simulink model "Project_Automotive_Performance_Modes"  (R2023a)
settings: Solver=VariableStepAuto  StartTime=0.0  StopTime=10.0  RelTol=1e-3
libraries: simulink x3, SignalEditorBlockLib x1
settings Model: Creator=Aman  LastModifiedBy=Aman

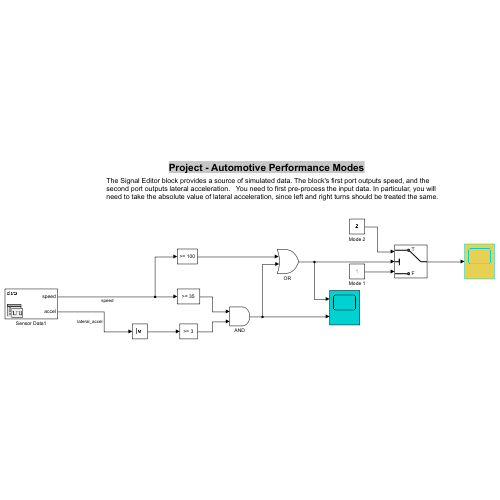
[thumbnail: Simulink's stored preview of the top-level diagram]
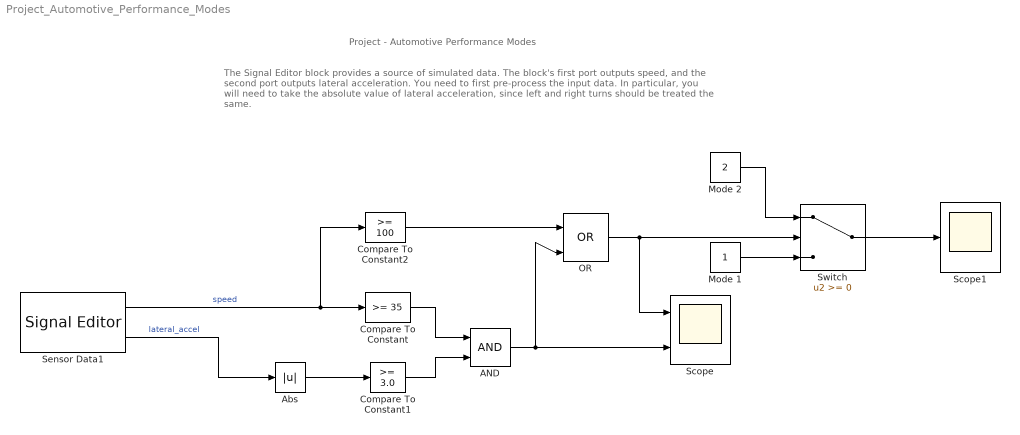
== system Project_Automotive_Performance_Modes ==
  note: The Signal Editor block provides a source of simulated data. The block's first port outputs speed, and the second port outputs lateral acceleration. You need to first pre-process the input data. In particular, you will need to take the absolute value of lateral acceleration, since left and right turns should be treated the same.
  note: Project - Automotive Performance Modes
  AND : Logic  IconShape=distinctive  AllPortsSameDT=off  OutDataTypeStr=boolean
  Abs : Abs  SaturateOnIntegerOverflow=off
  Compare To Constant : simulink/Logic and Bit Operations/Compare To Constant  relop=>=  const=35  OutDataTypeStr=boolean
  Compare To Constant1 : simulink/Logic and Bit Operations/Compare To Constant  relop=>=  const=3.0  OutDataTypeStr=boolean
  Compare To Constant2 : simulink/Logic and Bit Operations/Compare To Constant  relop=>=  const=100  OutDataTypeStr=boolean
  Mode 1 : Constant
  Mode 2 : Constant  Value=2
  OR : Logic  Operator=OR  IconShape=distinctive  AllPortsSameDT=off  OutDataTypeStr=boolean
  Scope : Scope  NumInputPorts=2
  Scope1 : Scope
  Sensor Data1 : SignalEditorBlockLib/Signal Editor  FileName=signalData.mat  ActiveScenario=data  ActiveSignal=speed  IsBus=off  OutputBusObjectStr=Bus: BusObject  SampleTime=0  Interpolate=off  ZeroCross=off  OutputAfterFinalValue=Setting to zero  Unit=inherit  PreserveSignalName=on  ApplySigPropsToAllScenarios=on
  Switch : Switch  SaturateOnIntegerOverflow=off  InputSameDT=off
  wires:
  Sensor Data1/1 -> Compare To Constant2/1, Compare To Constant/1  "speed"
  Compare To Constant/1 -> AND/1
  Compare To Constant1/1 -> AND/2
  Sensor Data1/2 -> Abs/1  "lateral_accel"
  Abs/1 -> Compare To Constant1/1
  AND/1 -> Scope/2, OR/2
  Compare To Constant2/1 -> OR/1
  OR/1 -> Scope/1, Switch/2
  Mode 2/1 -> Switch/1
  Mode 1/1 -> Switch/3
  Switch/1 -> Scope1/1
